simulink model "Temperature_Estimation"  (R2024a)
settings: Solver=VariableStepAuto  StartTime=0.0  StopTime=10.0  RelTol=1e-3
settings Model: Creator=ACER  LastModifiedBy=ACER

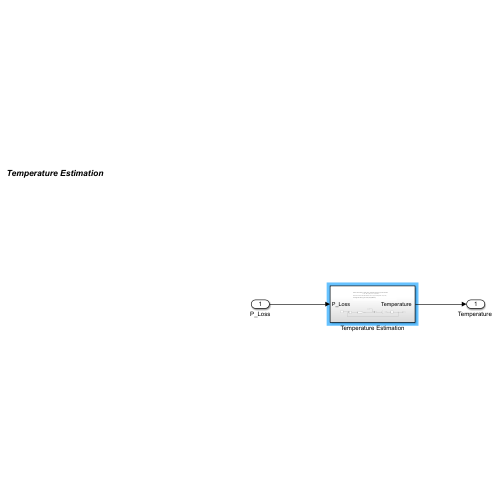
[thumbnail: Simulink's stored preview of the top-level diagram]
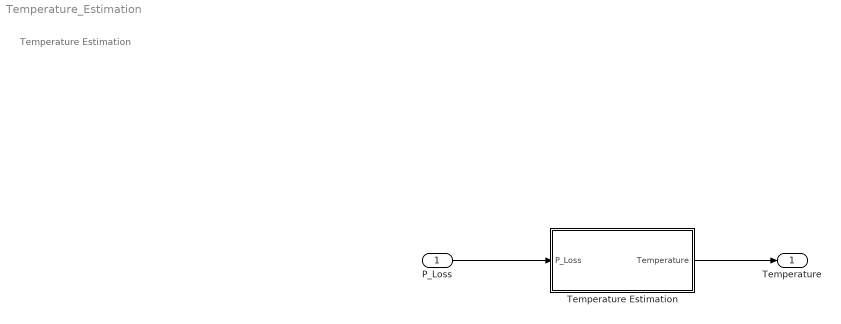
== system Temperature_Estimation ==
  note: Temperature Estimation
  P_Loss : Inport
  Temperature Estimation : Subsystem
  "Temperature " : Outport
  wires:
  P_Loss/1 -> Temperature Estimation/1(P_Loss)
  Temperature Estimation/1("Temperature ") -> "Temperature "/1

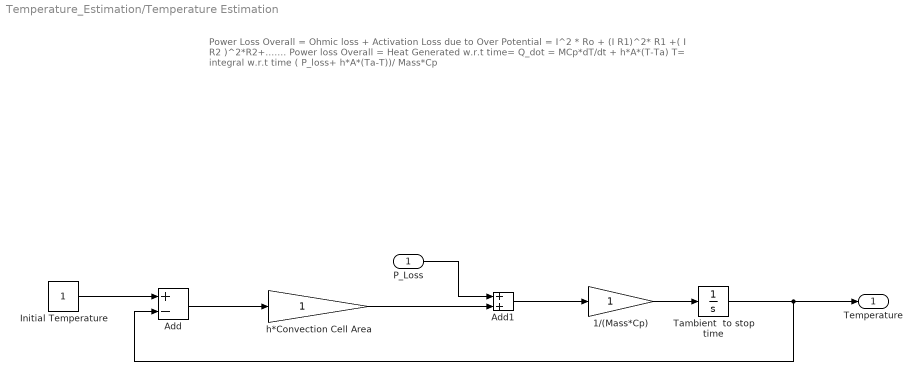
== system Temperature_Estimation/Temperature Estimation ==
  note: Power Loss Overall = Ohmic loss + Activation Loss due to Over Potential
      | = I^2 * Ro + (I R1)^2* R1 +( I R2 )^2*R2+.......
      |
      | Power loss Overall = Heat Generated w.r.t time= Q_dot = MCp*dT/dt + h*A*(T-Ta)
      |
      | T= integral w.r.t time ( P_loss+ h*A*(Ta-T))/ Mass*Cp
  P_Loss : Inport
  1/(Mass*Cp) : Gain
  Add : Sum  Inputs=+-
  Add1 : Sum
  "Initial Temperature " : Constant
  Tambient  to stop time : Integrator
  "h*Convection Cell Area " : Gain
  "Temperature " : Outport
  wires:
  Tambient  to stop time/1 -> "Temperature "/1, Add/2
  "h*Convection Cell Area "/1 -> Add1/2
  Add/1 -> "h*Convection Cell Area "/1
  "Initial Temperature "/1 -> Add/1
  Add1/1 -> 1/(Mass*Cp)/1
  P_Loss/1 -> Add1/1
  1/(Mass*Cp)/1 -> Tambient  to stop time/1
